simulink model "homerseklet"  (Simulink 8.1)
settings: Solver=ode45  StartTime=0.0  StopTime=80  RelTol=1e-3
settings Model: Creator=Rudi  LastModifiedBy=rudi

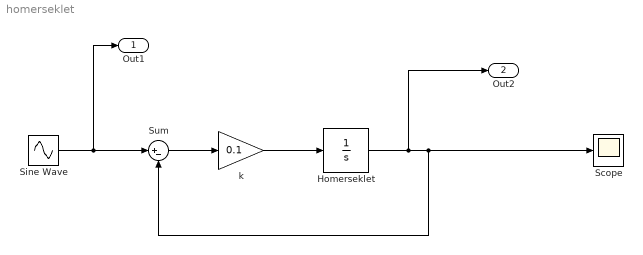
== system homerseklet ==
  Homerseklet : Integrator  InitialCondition=20
  Scope : Scope
  Sine Wave : Sin  Amplitude=10  Bias=100  Frequency=0.5  SampleTime=0
  Sum : Sum  Inputs=|+-
  k : Gain  Gain=0.1
  Out1 : Outport
  Out2 : Outport  Port=2
  wires:
  Homerseklet/1 -> Sum/2, Scope/1, Out2/1
  Sum/1 -> k/1
  k/1 -> Homerseklet/1
  Sine Wave/1 -> Sum/1, Out1/1
